simulink model "PPM"  (R2020a)
settings: Solver=VariableStepAuto  StartTime=0.0  StopTime=10.0  RelTol=1e-3
libraries: dspsrcs4 x1, dspswit3 x1, dspsigops x1
settings Model: Creator=jeeva  LastModifiedBy=jeeva

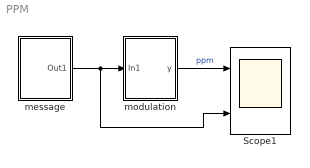
== system PPM ==
  Scope1 : Scope  NumInputPorts=2
  message : Subsystem
  modulation : Subsystem
  wires:
  message/1(Out1) -> Scope1/2, modulation/1(In1)
  modulation/1(y) -> Scope1/1  "ppm"

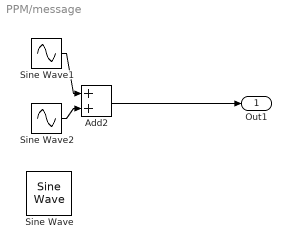
== system PPM/message ==
  Add2 : Sum
  Sine Wave : dspsrcs4/Sine Wave  Amplitude=1  Frequency=100  Phase=0  SampleMode=Discrete  OutComplex=Real  CompMethod=Trigonometric fcn  TableSize=Speed  SampleTime=1/1000  SamplesPerFrame=1  ResetState=Restart at time zero  OutputFrames=off  dataType=double  wordLen=16  udDataType=sfix(16)  fracBitsMode=Best precision  numFracBits=15  OutDataTypeStr=double  LastOutDataTypeStr=double
  Sine Wave1 : Sin  Amplitude=0.7  Frequency=2  SampleTime=0
  Sine Wave2 : Sin  Amplitude=0.5  Frequency=1.5  SampleTime=0
  Out1 : Outport
  wires:
  Sine Wave2/1 -> Add2/2
  Sine Wave1/1 -> Add2/1
  Add2/1 -> Out1/1

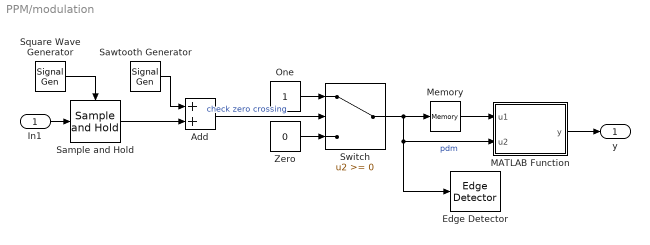
== system PPM/modulation ==
  In1 : Inport
  Add : Sum
  Edge Detector : dspswit3/Edge Detector  InputProcessing=Columns as channels (frame based)
      settings: SourceProductBaseCode=DS
  MATLAB Function : MATLAB Function  TreatAsAtomicUnit=on
  Memory : Memory  InheritSampleTime=on
  One : Constant  OutDataTypeStr=Inherit: Inherit via back propagation
  Sample and Hold : dspsigops/Sample and Hold  trig=Rising edge  initCond=0  latchinput=off
  Sawtooth Generator : SignalGenerator  WaveForm=sawtooth  Amplitude=2  Frequency=4
  Square Wave Generator : SignalGenerator  WaveForm=square  Frequency=2
  Switch : Switch
  Zero : Constant  Value=0  OutDataTypeStr=Inherit: Inherit via back propagation
  y : Outport
  wires:
  Zero/1 -> Switch/3
  Sawtooth Generator/1 -> Add/1
  Memory/1 -> MATLAB Function/1(u1)
  Switch/1 -> Edge Detector/1, MATLAB Function/2(u2), Memory/1  "pdm"
  Sample and Hold/1 -> Add/2
  Square Wave Generator/1 -> Sample and Hold/Trigger
  Add/1 -> Switch/2  "check zero crossing"
  One/1 -> Switch/1
  In1/1 -> Sample and Hold/1
  MATLAB Function/1(y) -> y/1

== matlab function PPM/modulation/MATLAB Function ==
  data: u1 input; y output; u2 input
function y = fcn(u1, u2)
if (u1 == u2)
    y = 0;
else 
    y = 1;
end
